simulink model "model"  (R2025b)
settings: Solver=VariableStepAuto  StartTime=0.0  StopTime=50  RelTol=1e-3
values from neighbouring files (symbols this model uses):
  a = 0.1165    [model_init.m]
  b = -3.915    [model_init.m]
  c = -0.008    [model_init.m]
  d = 0.00229    [model_init.m]
  J = 0.000115    [model_init.m]
  K = lqr(A, B, Q, R)    [model_init.m]
  Km = 484.73    [model_init.m]
  Ks = 1    [model_init.m]
  mgl = 4    [model_init.m]
  SP = [pi, 0, 0]    [model_init.m]
  x0 = [0.1 ; 6; 0]    [model_init.m]
settings Model: Creator=kamil  LastModifiedBy=filip
settings SolverCC: ZeroCrossAlgorithm=Adaptive
settings DebuggingCC: IgnoredZcDiagnostic=none

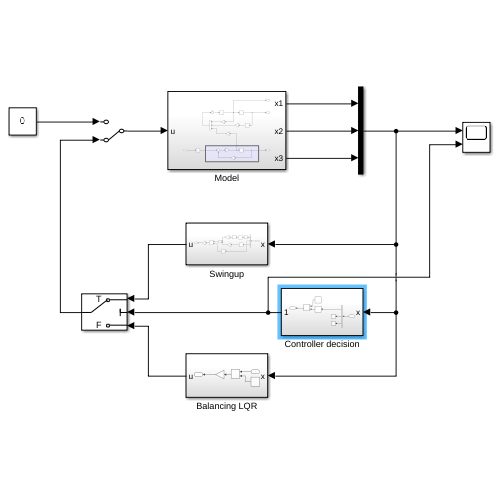
[thumbnail: Simulink's stored preview of the top-level diagram]
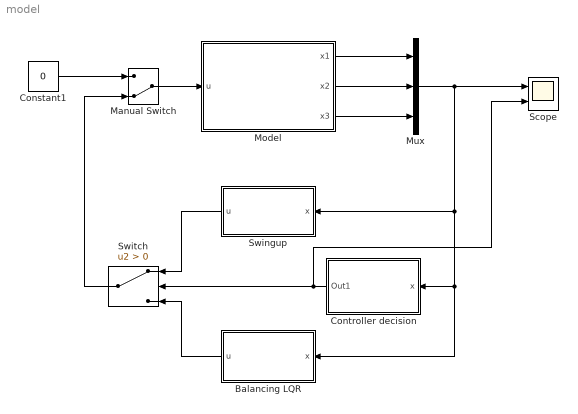
== system model ==
  Balancing LQR : Subsystem
  Constant1 : Constant  Value=0
  Controller decision : Subsystem
  Manual Switch : ManualSwitch  CurrentSetting=0
  Model : Subsystem
  Mux : Mux  Inputs=3
  Scope : Scope  NumInputPorts=2
      settings: ActiveDisplayYMinimum=-16.473284026248997  ActiveDisplayYMaximum=13.861975296147758
  Swingup : Subsystem
  Switch : Switch  Criteria=u2 > Threshold  SaturateOnIntegerOverflow=off  InputSameDT=off
  wires:
  Model/2(x2) -> Mux/2
  Manual Switch/1 -> Model/1(u)
  Constant1/1 -> Manual Switch/1
  Model/1(x1) -> Mux/1
  Balancing LQR/1(u) -> Switch/3
  Swingup/1(u) -> Switch/1
  Switch/1 -> Manual Switch/2
  Model/3(x3) -> Mux/3
  Controller decision/1(Out1) -> Scope/2, Switch/2
  Mux/1 -> Controller decision/1(x), Balancing LQR/1(x), Swingup/1(x), Scope/1

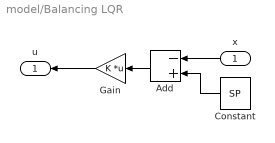
== system model/Balancing LQR ==
  x : Inport
  Add : Sum  Inputs=-+
  Constant : Constant  Value=SP
  Gain : Gain  Gain=K  Multiplication=Matrix(K*u)
  u : Outport
  wires:
  Add/1 -> Gain/1
  x/1 -> Add/1
  Gain/1 -> u/1
  Constant/1 -> Add/2

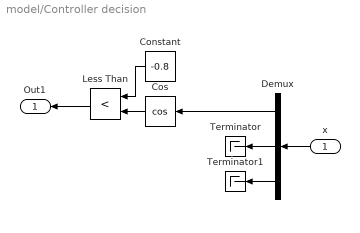
== system model/Controller decision ==
  x : Inport
  Constant : Constant  Value=-0.8
  Cos : Trigonometry  Operator=cos
  Demux : Demux  Outputs=3
  Less Than : RelationalOperator  Operator=<  OutDataTypeStr=boolean  RndMeth=Simplest  InputSameDT=off
  Terminator : Terminator
  Terminator1 : Terminator
  Out1 : Outport
  wires:
  Constant/1 -> Less Than/1
  Cos/1 -> Less Than/2
  Less Than/1 -> Out1/1
  Demux/1 -> Cos/1
  x/1 -> Demux/1
  Demux/2 -> Terminator/1
  Demux/3 -> Terminator1/1

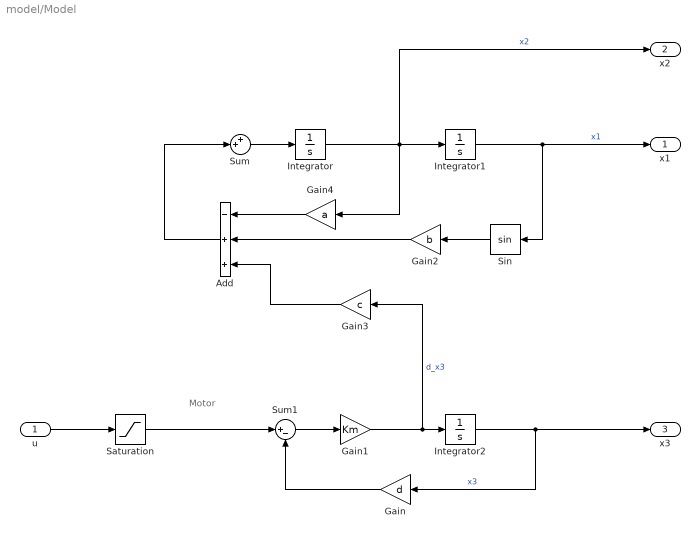
== system model/Model ==
  note: Motor
  u : Inport
  Add : Sum  Inputs=-++
  Gain : Gain  Gain=d
  Gain1 : Gain  Gain=Km
  Gain2 : Gain  Gain=b
  Gain3 : Gain  Gain=c
  Gain4 : Gain  Gain=a
  Integrator : Integrator  InitialCondition=x0(2)
  Integrator1 : Integrator  InitialCondition=x0(1)
  Integrator2 : Integrator  InitialCondition=x0(3)
  Saturation : Saturate  UpperLimit=1  LowerLimit=-1
  Sin : Trigonometry
  Sum : Sum  Inputs=++|
  Sum1 : Sum  Inputs=|+-
  x1 : Outport
  x2 : Outport  Port=2
  x3 : Outport  Port=3
  wires:
  Sin/1 -> Gain2/1
  Gain3/1 -> Add/3
  Sum1/1 -> Gain1/1
  Integrator1/1 -> x1/1, Sin/1  "x1"
  Gain4/1 -> Add/1
  Add/1 -> Sum/2
  Gain2/1 -> Add/2
  Integrator/1 -> x2/1, Integrator1/1, Gain4/1  "x2"
  Gain1/1 -> Gain3/1, Integrator2/1  "d_x3"
  Gain/1 -> Sum1/2
  Integrator2/1 -> x3/1, Gain/1  "x3"
  u/1 -> Saturation/1
  Saturation/1 -> Sum1/1
  Sum/1 -> Integrator/1

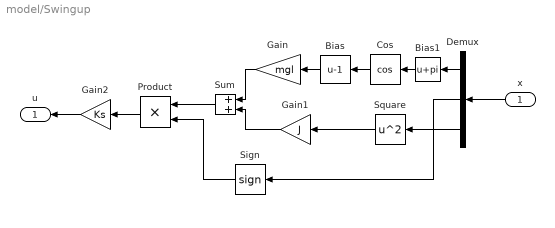
== system model/Swingup ==
  x : Inport
  Bias : Bias  Bias=-1  SaturateOnIntegerOverflow=off
  Bias1 : Bias  Bias=pi  SaturateOnIntegerOverflow=off
  Cos : Trigonometry  Operator=cos
  Demux : Demux  Outputs=3
  Gain : Gain  Gain=mgl
  Gain1 : Gain  Gain=J
  Gain2 : Gain  Gain=Ks
  Product : Product
  Sign : Signum
  Square : Math  Operator=square
  Sum : Sum
  u : Outport
  wires:
  x/1 -> Demux/1
  Cos/1 -> Bias/1
  Product/1 -> Gain2/1
  Demux/3 -> Square/1
  Demux/2 -> Sign/1
  Sum/1 -> Product/1
  Gain1/1 -> Sum/2
  Sign/1 -> Product/2
  Demux/1 -> Bias1/1
  Gain/1 -> Sum/1
  Square/1 -> Gain1/1
  Bias1/1 -> Cos/1
  Gain2/1 -> u/1
  Bias/1 -> Gain/1
